simulink model "smo_pmsm"  (R2014a)
settings: Solver=ode45  StartTime=0.0  StopTime=0.5  RelTol=1e-3
InitFcn:
  | parameter
undefined symbols (not defined in the file): DiscIntNeverNeededParam, fc1, K, ki_i, ki_pll, ki_v, kp_i, kp_pll, kp_v, L, powergui, R, sigbuilder_block, Threshold, TS, Vdc, wc
libraries: powerlib x3, simulink x2, AC6DriveInternalModels x1
Description:
  | parameter.m;
settings Model: Creator=jzj  LastModifiedBy=jzj
settings ModelReferenceCC: ModelDependencies=parameter.m;

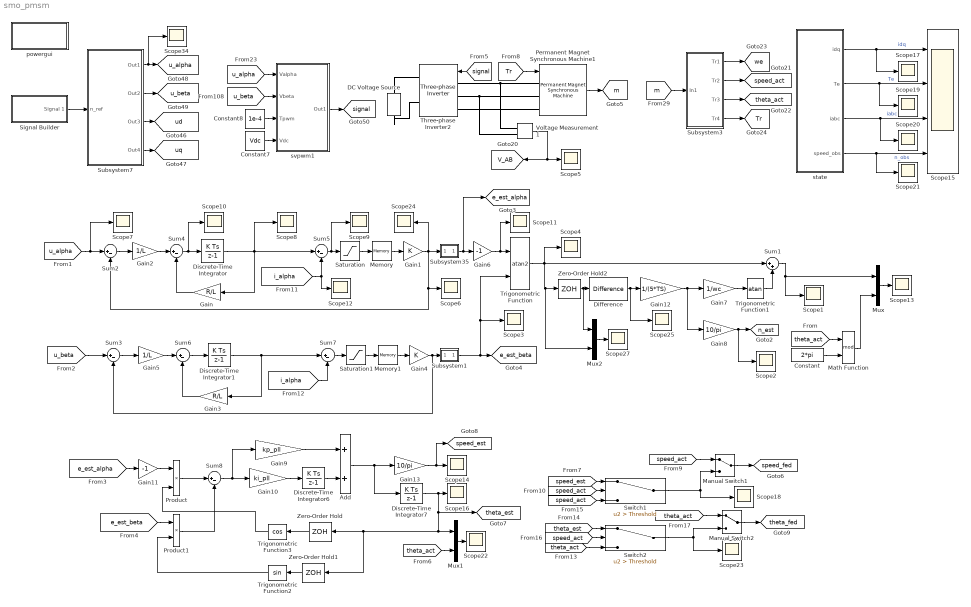
== system smo_pmsm ==
  Add : Sum
  Constant : Constant  Value=2*pi
  Constant7 : Constant  Value=Vdc
  Constant8 : Constant  Value=1e-4
  DC Voltage Source : powerlib/Electrical Sources/DC Voltage Source  Amplitude=Vdc  Measurements=Voltage
  Difference : simulink/Discrete/Difference  ICPrevInput=0.0  InputProcessing=Inherited  OutMin=[]  OutMax=[]  OutDataType=fixdt(1, 16)  OutScaling=2^-10  DoSatur=off
  Discrete-Time Integrator{,1,6..7} (4 alike) : DiscreteIntegrator  SampleTime=-1  ICPrevOutput=DiscIntNeverNeededParam  ICPrevScaledInput=DiscIntNeverNeededParam
  Gain : Gain  Gain=R/L
  Gain1 : Gain  Gain=K
  Gain10 : Gain  Gain=ki_pll
  Gain11 : Gain  Gain=-1
  Gain12 : Gain  Gain=1/(5*TS)
  Gain13 : Gain  Gain=10/pi
  Gain2 : Gain  Gain=1/L
  Gain3 : Gain  Gain=R/L
  Gain4 : Gain  Gain=K
  Gain5 : Gain  Gain=1/L
  Gain6 : Gain  Gain=-1
  Gain7 : Gain  Gain=1/wc
  Gain8 : Gain  Gain=10/pi
  Gain9 : Gain  Gain=kp_pll
  Manual Switch1 : ManualSwitch
  Manual Switch2 : ManualSwitch
  Math Function : Math  Operator=mod  SaturateOnIntegerOverflow=on
  Memory : Memory  InheritSampleTime=on
  Memory1 : Memory  InheritSampleTime=on
  Mux : Mux  Inputs=2
  Mux1 : Mux  Inputs=2
  Mux2 : Mux  Inputs=2
  Permanent Magnet Synchronous Machine1 : powerlib/Machines/Permanent Magnet Synchronous Machine  NbPhases=3  FluxDistribution=Sinusoidal  RotorType=Round  MechanicalLoad=Torque Tm  PresetModel=No  ShowDetailedParameters=on  MeasurementBus=off  Resistance=0.8  Inductance=0  dqInductances=[0.01,0.02]  La=0.0012  MachineConstant=Voltage Constant (V_peak L-L / krpm)  Flux=0.003308  VoltageCst=2.4  TorqueCst=0.019848  Flat=0  Mechanical=[0.0001,0,4]  PolePairs=3  InitialConditions=[0,0, 0,0]  InitialConditions5ph=[0 0 0 0 0 0]  TsPowergui=0  TsBlock=-1  RefAngle=Aligned with phase A axis (original Park)
      link override From: GotoTag=tp24d3e2ed_e96a_4fb0_a076_5c3b1daf5e05
      settings: AttributesFormatString=\n
  Product : Product
  Product1 : Product
  Saturation : Saturate  UpperLimit=5  LowerLimit=-5
  Saturation1 : Saturate  UpperLimit=5  LowerLimit=-5
  Scope{1..14,16..25,27,34} (26 alike) : Scope
      Scope1 settings: YMin=-700  YMax=700  SaveName=ScopeData7
      Scope10 settings: YMin=-700  YMax=700  SaveName=ScopeData24
      Scope11 settings: YMin=-700  YMax=700  SaveName=ScopeData25
      Scope12 settings: YMin=-700  YMax=700  SaveName=ScopeData31
      Scope13 settings: YMin=-700  YMax=700  SaveName=ScopeData32
      Scope14 settings: YMin=-700  YMax=700  SaveName=ScopeData33
      Scope16 settings: YMin=-700  YMax=700  SaveName=ScopeData34
      Scope17 settings: YMin=-700  YMax=700  SaveName=ScopeData18
      Scope18 settings: YMin=-700  YMax=700  SaveName=ScopeData35
      Scope19 settings: YMin=-700  YMax=700  SaveName=ScopeData19
      Scope2 settings: YMin=-700  YMax=700  SaveName=ScopeData10
      Scope20 settings: YMin=-700  YMax=700
      Scope21 settings: TimeRange=3  YMin=4200  YMax=5500  SaveName=ScopeData4
      Scope22 settings: YMin=-700  YMax=700  SaveName=ScopeData36
      Scope23 settings: YMin=-700  YMax=700  SaveName=ScopeData39
      Scope24 settings: YMin=-700  YMax=700  SaveName=ScopeData40
      Scope25 settings: YMin=-700  YMax=700  SaveName=ScopeData41
      Scope27 settings: YMin=-700  YMax=700  SaveName=ScopeData43
      Scope3 settings: YMin=-700  YMax=700  SaveName=ScopeData11
      Scope34 settings: YMin=-700  YMax=700  SaveName=ScopeData38
      Scope4 settings: YMin=-700  YMax=700  SaveName=ScopeData13
      Scope5 settings: YMin=-700  YMax=700  SaveName=ScopeData78
      Scope6 settings: YMin=-700  YMax=700  SaveName=ScopeData14
      Scope7 settings: YMin=-700  YMax=700  SaveName=ScopeData15
      Scope8 settings: YMin=-700  YMax=700  SaveName=ScopeData16
      Scope9 settings: YMin=-700  YMax=700  SaveName=ScopeData17
  Scope15 : Scope  NumInputPorts=4
      settings: TimeRange=1.5  YMin=-17.5~-5~-80~-400  YMax=15~35~60~900  SaveName=ScopeData20
  Signal Builder : Subsystem  Tag=STV Subsys  LoadFcn=sigbuilder_block('load');  StartFcn=sigbuilder_block('start');  StopFcn=sigbuilder_block('stop');  ClipboardFcn=sigbuilder_block('clipboard');  mask(Sigbuilder block){}
      mask help: Simulink:masks:SigbuilderBlock_MD
      mask init:
      | if ~strcmp(get_param(bdroot(gcbh),'SimulationStatus'),'stopped') tuvar = sigbuilder_block('maskInit'); end
      settings: CopyFcn=sigbuilder_block('copy');  DeleteFcn=sigbuilder_block('delete');  ModelCloseFcn=sigbuilder_block('modelClose');  PreSaveFcn=sigbuilder_block('preSave');  PauseFcn=sigbuilder_block('pause');  ContinueFcn=sigbuilder_block('continue');  NameChangeFcn=sigbuilder_block('namechange');  OpenFcn=sigbuilder_block('open',[497.25 145.5 550.5 399.75 ]);  CloseFcn=sigbuilder_block('close');
      mask Display: plot(0, 0, 100, 100,[2, 2, 32, 32, 2], [68, 8, 8, 68, 68],[32, 2], [38, 38], [32, 19, 2],[53, 60, 44], [32, 17, 17, 2],[16, 16, 31, 31]);txt = getActiveGroup(gcbh);text(2, 100, txt,'verticalAlignment', 'top');
  Subsystem1 : Subsystem
  Subsystem3 : Subsystem
  Subsystem35 : Subsystem
  Subsystem7 : Subsystem
  Sum1 : Sum  Inputs=|++
  Sum{2..8} (7 alike) : Sum  Inputs=|+-
  Switch1 : Switch  Criteria=u2 > Threshold  Threshold=Threshold
  Switch2 : Switch  Criteria=u2 > Threshold  Threshold=Threshold
  Three-phase Inverter2 : AC6DriveInternalModels/Three-phase Inverter  Arms=3  SnubberResistance=5000  SnubberCapacitance=inf  Device=IGBT / Diodes  Ron=1e-3  Lon=0  ForwardVoltages=[0.8,0.8]  ForwardVoltage=0  GTOparameters=[0,0]  IGBTParameters=[1e-6,2e-6]  Measurements=All voltages and currents  converterType=Inverter  SourceFrequency=60  dqInductances=[8.5e-3,8.5e-3]  Flux=0.175  Resistance=0.2  p=4
  Trigonometric Function : Trigonometry  Operator=atan2
  Trigonometric Function1 : Trigonometry  Operator=atan
  Trigonometric Function2 : Trigonometry
  Trigonometric Function3 : Trigonometry  Operator=cos
  Voltage Measurement1 : powerlib/Measurements/Voltage Measurement  PhasorSimulation=off  OutputType=Complex  PSBequivalent=0
  Zero-Order Hold : ZeroOrderHold  SampleTime=TS
  Zero-Order Hold1 : ZeroOrderHold  SampleTime=TS
  Zero-Order Hold2 : ZeroOrderHold  SampleTime=5*TS
  powergui : Subsystem  Priority=1  AncestorBlock=powerlib/powergui  InitFcn=powergui( 'InitFcn_Callback' , gcb , 0 , [ ] );  StopFcn=powergui( 'StopFcn_Callback' , gcb , 0 , [ ] );  mask(PSB option menu block){SimulationMode=Discrete, SolverType=Tustin, SampleTime=1e-6, frequency=60, SPID=off, DisableSnubberDevices=off, DisableRonSwitches=off, DisableVfSwitches=off, SwTol=0, Interpol=off, DisplayEquations=off, Ts=100, methode=off, frequencyindice=0, Pbase=100e6, ErrMax=1e-4, Iterations=50, UnitsV=kV, UnitsW=MW, FunctionMessages=off, echomessages=off, HookPort=off, EnableUseOfTLC=off, x0status=blocks, RestoreLinks=warning, ResistiveCurrentMeasurement=off, Frange=[0:2:500], Ylog=off, Xlog=on, ShowGrid=off, save=off, variable=ZData, structure=iabc1, ZoomFFT=off, StartTime=2.2, cycles=50, DisplayStyle=1, fundamental=200, FreqAxis=on, MaxFrequency=500, frequencyindicesteady=1, RmsSteady=1, display=off}
      mask prompts: SimulationMode "Simulation type:"; SolverType "Solver type:"; SampleTime "Sample time (s):"; frequency "Phasor frequency (Hz):"; SPID "Enable use of ideal switching devices"; DisableSnubberDevices "Disable snubbers in switching devices"; DisableRonSwitches "Disable On resistance in switching devices (Ron=0)"; DisableVfSwitches "Disable Forward voltage in switching devices (Vf=0)"; SwTol "Switch tolerance"; Interpol "Interpolate"; DisplayEquations "Display circuit differential equations"; Ts "Old Ts setting (OBSOLETE)"; methode "Phasor simulation (OBSOLETE)"; frequencyindice "Load flow frequency (Hz):"; Pbase "Base power Pbase (VA):"; ErrMax "PQ tolerance (pu):"; Iterations "Max iterations:"; UnitsV "Voltage units"; UnitsW "Power units"; FunctionMessages "Disable SimPowerSystems warnings"; echomessages "Display SimPowerSystems compilation messages"; HookPort "Add a hook port to the powergui block"; EnableUseOfTLC "Use TLC file when in Accelerator Simulation Mode and for code generation"; x0status "Start simulation with initial electrical states from:"; RestoreLinks "Restore disabled links of SimPowerSystems blocks:"; ResistiveCurrentMeasurement "Use non ideal current measurement blocks (1e-4Ohm internal resistance)"; Frange "Frequency Range"; Ylog "Log impedance"; Xlog "log Frequency"; ShowGrid "grid"; save "Save Data To Workspace"; variable "Variable Name"; structure "Structure Name (PSBFFTSCOPE)"; ZoomFFT "ZoomFFT (PSBFFTSCOPE)"; StartTime "Start Time (PSBFFTSCOPE)"; cycles "Cycles (PSBFFTSCOPE)"; DisplayStyle "Display style (PSBFFTSCOPE)"; fundamental "Fundamental (PSBFFTSCOPE)"; FreqAxis "Frequency Axis (PSBFFTSCOPE)"; MaxFrequency "Max Frequency (PSBFFTSCOPE)"; frequencyindicesteady "Frequency indice (STEADYSTATE)"; RmsSteady "RMS display (STEADYSTATE)"; display "Display Results"
      mask help: Set simulation type, simulation parameters, and preferences
      mask init:
      | message = powergui('MaskInitialization',gcb,SimulationMode,SampleTime);
      settings: CopyFcn=powergui( 'Copy_Callback' , gcb , 0 , [ ] );  ModelCloseFcn=powergui( 'CloseButton_Callback' , gcb , [ ] , [ ] );  NameChangeFcn=powergui( 'NameChangeFcn_Callback' , gcb , 0 , [ ] );  OpenFcn=powergui(gcb,'Open')
      settings: DeleteFcn=|
      | % see geck 675031 powergui( 'Copy_Callback' , gcb , 1 , [ ] );
      | 
      | powergui( 'CloseButton_Callback' , gcb , [ ] , [ ] );
      settings: PreSaveFcn=|
      | powergui( 'PreSaveFcn_Callback' , gcb , [ ] , [ ] );
      | powergui( 'CloseButton_Callback' , gcb , [ ] , [ ] );
      mask Help: helpview(psbhelp)
      mask TypeOptions SimulationMode: Continuous | Discrete | Phasor
      mask Callback SimulationMode: powergui('SimulationType',[],[],gcb);
      mask TypeOptions SolverType: Tustin | Backward Euler
      mask Callback SPID: powergui('SPID',[],[],gcb);
      mask TypeOptions UnitsV: V | kV
      mask TypeOptions UnitsW: W | kW | MW
      mask Callback HookPort: powergui('HookPort',[],[],gcb);
      mask TypeOptions x0status: blocks | steady | zero
      mask TypeOptions RestoreLinks: yes | warning | no
      mask Display: color('blue'),disp(message)
  state : Subsystem
  svpwm1 : Subsystem
  tag scope: Tr=global, V_AB=global, e_est_alpha=global, e_est_beta=global, m=global, n_est=global, signal=global, speed_act=global, speed_est=global, speed_fed=global, theta_act=global, theta_est=global, theta_fed=global, u_alpha=global, u_beta=global, ud=global, uq=global, we=global
  wires:
  Subsystem7/1(Out1) -> [u_alpha], Scope34/1
  Subsystem7/2(Out2) -> [u_beta]
  Subsystem7/3(Out3) -> [ud]
  Subsystem7/4(Out4) -> [uq]
  Constant8/1 -> svpwm1/3(Tpwm)
  Constant7/1 -> svpwm1/4(Vdc)
  svpwm1/1(Out1) -> [signal]
  [u_alpha] -> svpwm1/1(Valpha)
  [u_beta] -> svpwm1/2(Vbeta)
  [signal] -> Three-phase Inverter2/1
  [Tr] -> Permanent Magnet Synchronous Machine1/1
  Permanent Magnet Synchronous Machine1/1 -> [m]
  Voltage Measurement1/1 -> [V_AB], Scope5/1
  [m] -> Subsystem3/1(In1)
  Subsystem3/1(Tr1) -> [we]
  Subsystem3/2(Tr2) -> [speed_act]
  Subsystem3/3(Tr3) -> [theta_act]
  Subsystem3/4(Tr4) -> [Tr]
  state/1(idq) -> Scope15/1, Scope17/1  "idq"
  state/2(Te) -> Scope15/2, Scope19/1  "Te"
  state/3(iabc) -> Scope15/3, Scope20/1  "iabc"
  state/4(speed_obs) -> Scope15/4, Scope21/1  "n_obs"
  Signal Builder/1(Signal 1) -> Subsystem7/1(n_ref)
  [u_beta] -> Sum3/1
  [u_alpha] -> Scope7/1, Sum2/1
  Sum2/1 -> Gain2/1
  Sum4/1 -> Scope10/1, Discrete-Time Integrator/1
  Gain/1 -> Sum4/2
  Discrete-Time Integrator/1 -> Scope8/1, Sum5/1, Gain/1
  [i_alpha] -> Scope12/1, Sum5/2
  Sum5/1 -> Scope9/1, Saturation/1
  Saturation/1 -> Memory/1
  Memory/1 -> Gain1/1
  Gain2/1 -> Sum4/1
  Sum6/1 -> Discrete-Time Integrator1/1
  Gain3/1 -> Sum6/2
  Discrete-Time Integrator1/1 -> Gain3/1, Sum7/1
  [i_alpha] -> Sum7/2
  Sum7/1 -> Saturation1/1
  Saturation1/1 -> Memory1/1
  Memory1/1 -> Gain4/1
  Gain5/1 -> Sum6/1
  Sum3/1 -> Gain5/1
  Gain1/1 -> Subsystem35/1(fil), Scope24/1, Scope6/1, Sum2/2
  Gain4/1 -> Subsystem1/1(fil), Sum3/2
  Subsystem35/1(ter) -> [e_est_alpha], Gain6/1
  Gain6/1 -> Scope11/1, Trigonometric Function/1
  Subsystem1/1(ter) -> [e_est_beta], Scope3/1, Trigonometric Function/2
  Trigonometric Function/1 -> Mux2/2, Zero-Order Hold2/1, Sum1/1, Scope4/1
  Gain7/1 -> Trigonometric Function1/1
  Trigonometric Function1/1 -> Sum1/2
  Sum1/1 -> Scope1/1, Mux/1
  Gain8/1 -> Scope2/1, [n_est]
  [theta_act] -> Math Function/1
  Constant/1 -> Math Function/2
  Math Function/1 -> Mux/2
  Mux/1 -> Scope13/1
  Discrete-Time Integrator6/1 -> Add/2
  Gain9/1 -> Add/1
  Gain10/1 -> Discrete-Time Integrator6/1
  [e_est_alpha] -> Gain11/1
  Gain11/1 -> Product/1
  [e_est_beta] -> Product1/1
  Product/1 -> Sum8/1
  Product1/1 -> Sum8/2
  Sum8/1 -> Gain9/1, Gain10/1
  Trigonometric Function3/1 -> Product/2
  Trigonometric Function2/1 -> Product1/2
  Discrete-Time Integrator7/1 -> [theta_est], Mux1/1, Zero-Order Hold1/1, Zero-Order Hold/1, Scope16/1
  Zero-Order Hold/1 -> Trigonometric Function3/1
  Zero-Order Hold1/1 -> Trigonometric Function2/1
  [theta_act] -> Mux1/2
  Mux1/1 -> Scope22/1
  Add/1 -> Discrete-Time Integrator7/1, Gain13/1
  Gain13/1 -> [speed_est], Scope14/1
  Manual Switch1/1 -> [speed_fed]
  [speed_act] -> Manual Switch1/1
  Switch1/1 -> Scope18/1, Manual Switch1/2
  [speed_act] -> Switch1/2
  [speed_act] -> Switch1/3
  [speed_est] -> Switch1/1
  [theta_est] -> Switch2/1
  [speed_act] -> Switch2/2
  [theta_act] -> Switch2/3
  Manual Switch2/1 -> [theta_fed]
  [theta_act] -> Manual Switch2/1
  Switch2/1 -> Manual Switch2/2, Scope23/1
  Zero-Order Hold2/1 -> Mux2/1, Difference/1
  Difference/1 -> Scope25/1, Gain12/1
  Gain12/1 -> Gain8/1, Gain7/1
  Mux2/1 -> Scope27/1
  connections:
  Three-phase Inverter2/LConn1 -- Permanent Magnet Synchronous Machine1/LConn1 -- Voltage Measurement1/LConn1
  Voltage Measurement1/LConn2 -- Permanent Magnet Synchronous Machine1/LConn2 -- Three-phase Inverter2/LConn2
  Permanent Magnet Synchronous Machine1/LConn3 -- Three-phase Inverter2/LConn3
  DC Voltage Source/RConn1 -- Three-phase Inverter2/RConn1
  DC Voltage Source/LConn1 -- Three-phase Inverter2/RConn2

== system smo_pmsm/Signal Builder ==
  Demux : Demux  Tag=STV Demux  Outputs=1
  FromWs : FromWorkspace  Tag=STV FromWs  VariableName=tuvar  SampleTime=0
      SigBuilderData=|
      | common.afterFinalStr = 'Extrapolate'
      | common.sampleTime = 0
      | dataSet.timeRange = [0 10]
      | dataSet.name = 'Group 1'
      | sbobj.Groups.Name = 'Group 1'
      | sbobj.Groups.Signals.Name = 'Signal 1'
      | sbobj.Groups.Signals.XData = [0 0.2 4 6 10]
      | sbobj.Groups.Signals.YData = [0 2000 2000 2000 2000]
  Signal 1 : Outport  Tag=STV Outport
  wires:
  Demux/1 -> Signal 1/1
  FromWs/1 -> Demux/1

== system smo_pmsm/Subsystem1 ==
  fil : Inport
  Low pass filter : DiscreteTransferFcn  Numerator=[1-exp(-2*pi*fc1*TS)]  Denominator=[1 -exp(-2*pi*fc1*TS)]  SampleTime=TS
  ter : Outport
  wires:
  Low pass filter/1 -> ter/1
  fil/1 -> Low pass filter/1

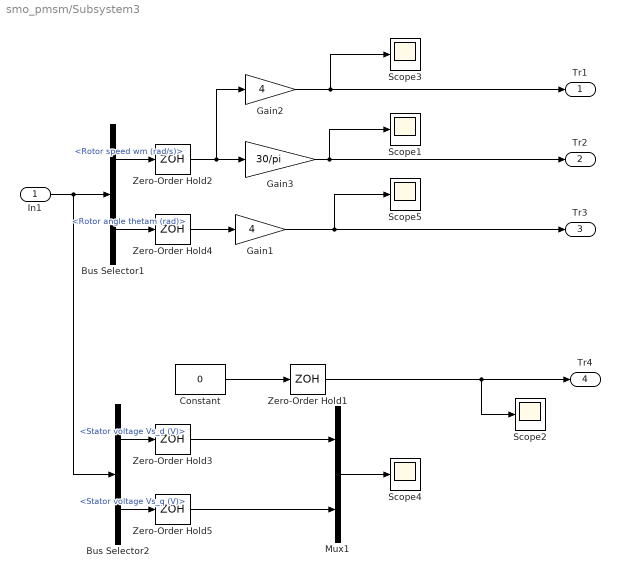
== system smo_pmsm/Subsystem3 ==
  In1 : Inport
  Bus Selector1 : BusSelector  OutputSignals=Rotor speed wm (rad/s),Rotor angle thetam (rad)
  Bus Selector2 : BusSelector  OutputSignals=Stator voltage Vs_d (V),Stator voltage Vs_q (V)
  Constant : Constant  Value=0
  Gain1 : Gain  Gain=4
  Gain2 : Gain  Gain=4
  Gain3 : Gain  Gain=30/pi
  Mux1 : Mux  Inputs=2
  Scope{1..5} (5 alike) : Scope
      Scope1 settings: YMin=-500  YMax=700  SaveName=ScopeData9
      Scope2 settings: YMin=-25  YMax=400  SaveName=ScopeData149
      Scope3 settings: YMin=185.5  YMax=191.5  SaveName=ScopeData79
      Scope4 settings: YMin=-25  YMax=400  SaveName=ScopeData88
      Scope5 settings: YMin=195  YMax=202.5  SaveName=ScopeData90
  Zero-Order Hold{1..5} (5 alike) : ZeroOrderHold  SampleTime=TS
  Tr1 : Outport
  Tr2 : Outport  Port=2
  Tr3 : Outport  Port=3
  Tr4 : Outport  Port=4
  wires:
  Zero-Order Hold5/1 -> Mux1/2
  Zero-Order Hold3/1 -> Mux1/1
  Constant/1 -> Zero-Order Hold1/1
  In1/1 -> Bus Selector1/1, Bus Selector2/1
  Bus Selector1/1 -> Zero-Order Hold2/1  "<Rotor speed wm (rad/s)>"
  Bus Selector1/2 -> Zero-Order Hold4/1  "<Rotor angle thetam (rad)>"
  Zero-Order Hold2/1 -> Gain2/1, Gain3/1
  Zero-Order Hold4/1 -> Gain1/1
  Gain2/1 -> Tr1/1, Scope3/1
  Gain3/1 -> Scope1/1, Tr2/1
  Zero-Order Hold1/1 -> Scope2/1, Tr4/1
  Bus Selector2/1 -> Zero-Order Hold3/1  "<Stator voltage Vs_d (V)>"
  Bus Selector2/2 -> Zero-Order Hold5/1  "<Stator voltage Vs_q (V)>"
  Gain1/1 -> Tr3/1, Scope5/1
  Mux1/1 -> Scope4/1

== system smo_pmsm/Subsystem35 ==
  fil : Inport
  Low pass filter : DiscreteTransferFcn  Numerator=[1-exp(-2*pi*fc1*TS)]  Denominator=[1 -exp(-2*pi*fc1*TS)]  SampleTime=TS
  ter : Outport
  wires:
  fil/1 -> Low pass filter/1
  Low pass filter/1 -> ter/1

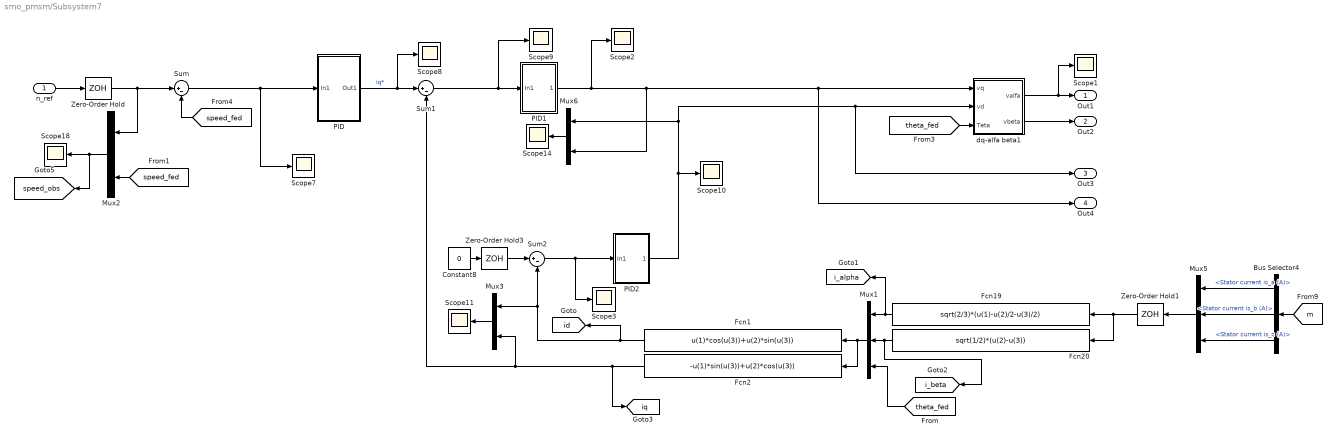
== system smo_pmsm/Subsystem7 ==
  n_ref : Inport
  Bus Selector4 : BusSelector  OutputSignals=Stator current is_a (A),Stator current is_b (A),Stator current is_c (A)
  Constant8 : Constant  Value=0
  Fcn1 : Fcn  Expr=u(1)*cos(u(3))+u(2)*sin(u(3))
  Fcn19 : Fcn  Expr=sqrt(2/3)*(u(1)-u(2)/2-u(3)/2)
  Fcn2 : Fcn  Expr=-u(1)*sin(u(3))+u(2)*cos(u(3))
  Fcn20 : Fcn  Expr=sqrt(1/2)*(u(2)-u(3))
  Mux1 : Mux  Inputs=3
  Mux2 : Mux  Inputs=2
  Mux3 : Mux  Inputs=2
  Mux5 : Mux  Inputs=3
  Mux6 : Mux  Inputs=2
  PID : Subsystem
  PID1 : Subsystem
  PID2 : Subsystem
  Scope{1..3,7..11,14,18} (10 alike) : Scope
      Scope1 settings: SaveName=ScopeData37
      Scope10 settings: SaveName=ScopeData30
      Scope11 settings: TimeRange=1.7  YMin=-15  YMax=17.5  SaveName=ScopeData71
      Scope14 settings: TimeRange=1.7  YMin=-15  YMax=17.5  SaveName=ScopeData106
      Scope18 settings: TimeRange=0.01073731461302402  YMin=996.9949713569969  YMax=1006.526183941498  SaveName=ScopeData21
      Scope2 settings: SaveName=ScopeData22
      Scope3 settings: SaveName=ScopeData23
      Scope7 settings: SaveName=ScopeData26
      Scope8 settings: SaveName=ScopeData28
      Scope9 settings: SaveName=ScopeData29
  Sum : Sum  Inputs=|+-
  Sum1 : Sum  Inputs=|+-
  Sum2 : Sum  Inputs=|+-
  Zero-Order Hold : ZeroOrderHold  SampleTime=TS
  Zero-Order Hold1 : ZeroOrderHold  SampleTime=TS
  Zero-Order Hold3 : ZeroOrderHold  SampleTime=TS
  dq-alfa beta1 : Subsystem
  Out1 : Outport
  Out2 : Outport  Port=2
  Out3 : Outport  Port=3
  Out4 : Outport  Port=4
  tag scope: i_alpha=global, i_beta=global, id=global, iq=global, speed_obs=global
  wires:
  Sum1/1 -> PID1/1(In1), Scope9/1
  Sum2/1 -> Scope3/1, PID2/1(In1)
  Mux2/1 -> [speed_obs], Scope18/1
  Sum/1 -> PID/1(In1), Scope7/1
  Constant8/1 -> Zero-Order Hold3/1
  Zero-Order Hold3/1 -> Sum2/1
  [theta_fed] -> dq-alfa beta1/3(Teta)
  [speed_fed] -> Mux2/2
  Zero-Order Hold/1 -> Sum/1, Mux2/1
  n_ref/1 -> Zero-Order Hold/1
  Mux3/1 -> Scope11/1
  PID/1(Out1) -> Scope8/1, Sum1/1  "iq*"
  [speed_fed] -> Sum/2
  PID2/1(Out1) -> Scope10/1, Mux6/1, dq-alfa beta1/2(vd), Out3/1
  PID1/1(Out1) -> Mux6/2, dq-alfa beta1/1(vq), Out4/1, Scope2/1
  dq-alfa beta1/1(valfa) -> Out1/1, Scope1/1
  dq-alfa beta1/2(vbeta) -> Out2/1
  Fcn1/1 -> Mux3/1, Sum2/2, [id]
  Fcn2/1 -> [iq], Sum1/2, Mux3/2
  Mux6/1 -> Scope14/1
  [m] -> Bus Selector4/1
  Bus Selector4/2 -> Mux5/2  "<Stator current is_b (A)>"
  Bus Selector4/3 -> Mux5/3  "<Stator current is_c (A)>"
  Bus Selector4/1 -> Mux5/1  "<Stator current is_a (A)>"
  Mux5/1 -> Zero-Order Hold1/1
  Fcn19/1 -> [i_alpha], Mux1/1
  Fcn20/1 -> [i_beta], Mux1/2
  [theta_fed] -> Mux1/3
  Mux1/1 -> Fcn2/1, Fcn1/1
  Zero-Order Hold1/1 -> Fcn20/1, Fcn19/1

== system smo_pmsm/powergui ==
  note: Graphical user interface for the analysis of  SimPowerSystems circuits.
      | Place the Powergui block in the top-level of your model and double-click
      | on it to open the GUI.
  EquivalentModel1 : Subsystem
      mask init:
      | S  = GetDataForEquivalentModel('Discrete',gcbh);
      mask Display:
      | color('red')
      | disp('EQUIVALENT CIRCUIT\nDiscrete')
  Ground : Ground
  Terminator : Terminator
  wires:
  Ground/1 -> Terminator/1

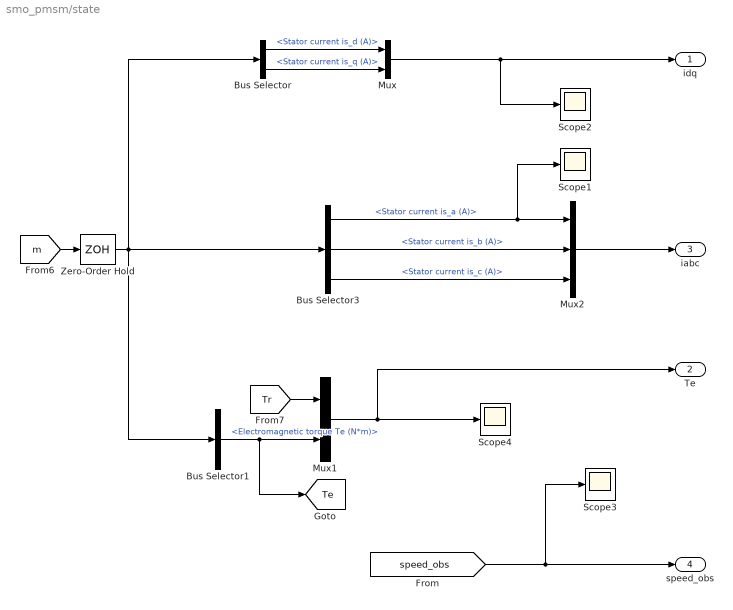
== system smo_pmsm/state ==
  Bus Selector : BusSelector  OutputSignals=Stator current is_d (A),Stator current is_q (A)
  Bus Selector1 : BusSelector  OutputSignals=Electromagnetic torque Te (N*m)
  Bus Selector3 : BusSelector  OutputSignals=Stator current is_a (A),Stator current is_b (A),Stator current is_c (A)
  Mux : Mux  Inputs=2
  Mux1 : Mux  Inputs=2
  Mux2 : Mux  Inputs=3
  Scope{1..4} (4 alike) : Scope
      Scope1 settings: TimeRange=0.7000000000000001  YMin=-4  YMax=8  SaveName=iabc
      Scope2 settings: TimeRange=0.7000000000000001  YMin=-2  YMax=18  SaveName=iabc1
      Scope3 settings: TimeRange=0.7000000000000001  YMin=1700  YMax=1712  SaveName=iabc2
      Scope4 settings: TimeRange=0.7000000000000001  YMin=-4  YMax=8  SaveName=iabc3
  Zero-Order Hold : ZeroOrderHold  SampleTime=TS
  idq : Outport
  Te : Outport  Port=2
  iabc : Outport  Port=3
  speed_obs : Outport  Port=4
  tag scope: Te=global
  wires:
  Bus Selector/1 -> Mux/1  "<Stator current is_d (A)>"
  Bus Selector/2 -> Mux/2  "<Stator current is_q (A)>"
  Bus Selector3/1 -> Mux2/1, Scope1/1  "<Stator current is_a (A)>"
  Bus Selector3/3 -> Mux2/3  "<Stator current is_c (A)>"
  Bus Selector3/2 -> Mux2/2  "<Stator current is_b (A)>"
  Bus Selector1/1 -> [Te], Mux1/2  "<Electromagnetic torque Te (N*m)>"
  [m] -> Zero-Order Hold/1
  [Tr] -> Mux1/1
  Mux/1 -> Scope2/1, idq/1
  Zero-Order Hold/1 -> Bus Selector/1, Bus Selector1/1, Bus Selector3/1
  Mux2/1 -> iabc/1
  [speed_obs] -> Scope3/1, speed_obs/1
  Mux1/1 -> Scope4/1, Te/1

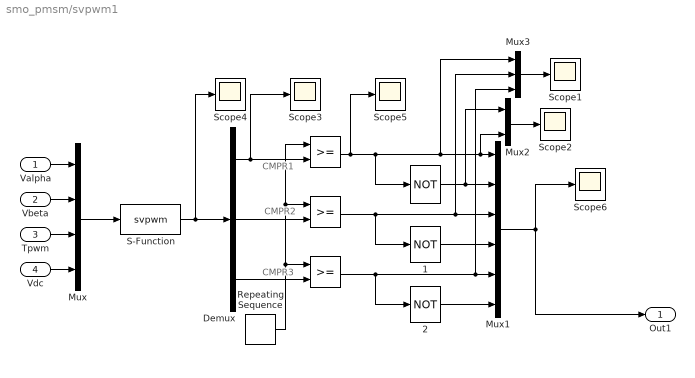
== system smo_pmsm/svpwm1 ==
  note: CMPR1
  note: CMPR2
  note: CMPR3
  Valpha : Inport
  Vbeta : Inport  Port=2
  Tpwm : Inport  Port=3
  Vdc : Inport  Port=4
  " " : RelationalOperator  ZeroCross=off
  "  " : RelationalOperator  OutDataTypeStr=boolean
  "   " : RelationalOperator  OutDataTypeStr=boolean
  "    " : Logic  Operator=NOT  Inputs=1  AllPortsSameDT=off  OutDataTypeStr=boolean
  "    1" : Logic  Operator=NOT  Inputs=1  AllPortsSameDT=off  OutDataTypeStr=boolean
  "    2" : Logic  Operator=NOT  Inputs=1  AllPortsSameDT=off  OutDataTypeStr=boolean
  Demux : Demux  Outputs=3
  Mux : Mux
  Mux1 : Mux  Inputs=6
  Mux2 : Mux  Inputs=2
  Mux3 : Mux  Inputs=3
  Repeating Sequence : simulink/Sources/Repeating Sequence  rep_seq_t=[0 0.00005 0.0001]  rep_seq_y=[0 0.00005 0]
  S-Function : S-Function  FunctionName=svpwm  EnableBusSupport=off
  Scope{1..6} (6 alike) : Scope
      Scope1 settings: TimeRange=1  YMin=-1  YMax=2  SaveName=ScopeData3
      Scope2 settings: TimeRange=0.2  YMin=-2.5e-006  YMax=5.25e-005  SaveName=ScopeData5
      Scope3 settings: TimeRange=0.2  YMin=-2.5e-006  YMax=5.25e-005
      Scope4 settings: TimeRange=0.2  YMin=-2.5e-006  YMax=5.25e-005  SaveName=ScopeData6
      Scope5 settings: TimeRange=0.2  YMin=-2.5e-006  YMax=5.25e-005  SaveName=ScopeData2
      Scope6 settings: TimeRange=0.2  YMin=-2.5e-006  YMax=5.25e-005  SaveName=ScopeData8
  Out1 : Outport
  wires:
  Demux/1 -> " "/2, Scope3/1
  Demux/2 -> "  "/2
  Demux/3 -> "   "/2
  "   "/1 -> "    2"/1, Mux1/5, Mux3/3
  "    "/1 -> Mux1/2, Mux2/1
  " "/1 -> Mux1/1, Mux2/2, Mux3/1, "    "/1, Scope5/1
  "  "/1 -> "    1"/1, Mux1/3, Mux3/2
  "    1"/1 -> Mux1/4
  "    2"/1 -> Mux1/6
  Repeating Sequence/1 -> "  "/1, " "/1, "   "/1
  S-Function/1 -> Demux/1, Scope4/1
  Valpha/1 -> Mux/1
  Vbeta/1 -> Mux/2
  Tpwm/1 -> Mux/3
  Vdc/1 -> Mux/4
  Mux3/1 -> Scope1/1
  Mux/1 -> S-Function/1
  Mux1/1 -> Out1/1, Scope6/1
  Mux2/1 -> Scope2/1

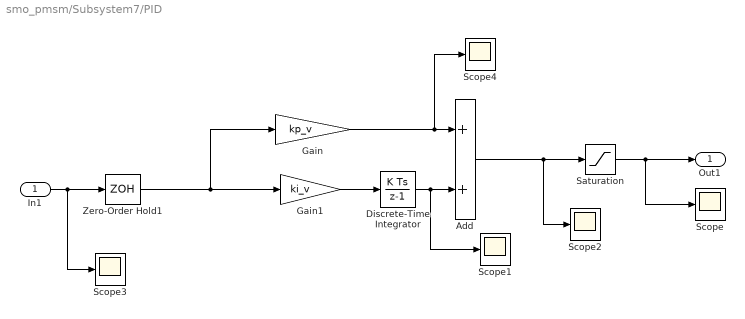
== system smo_pmsm/Subsystem7/PID ==
  In1 : Inport
  Add : Sum
  Discrete-Time Integrator : DiscreteIntegrator  InitialConditionSetting=State (most efficient)  SampleTime=-1  ICPrevOutput=DiscIntNeverNeededParam  ICPrevScaledInput=DiscIntNeverNeededParam
  Gain : Gain  Gain=kp_v
  Gain1 : Gain  Gain=ki_v
  Saturation : Saturate  UpperLimit=15  LowerLimit=-10
  Scope{,1..4} (5 alike) : Scope
      Scope settings: SaveName=ScopeData12
      Scope1 settings: SaveName=ScopeData27
      Scope2 settings: SaveName=ScopeData68
      Scope3 settings: SaveName=ScopeData69
      Scope4 settings: SaveName=ScopeData87
  Zero-Order Hold1 : ZeroOrderHold  SampleTime=TS
  Out1 : Outport
  wires:
  In1/1 -> Scope3/1, Zero-Order Hold1/1
  Gain/1 -> Scope4/1, Add/1
  Discrete-Time Integrator/1 -> Scope1/1, Add/2
  Add/1 -> Scope2/1, Saturation/1
  Saturation/1 -> Out1/1, Scope/1
  Gain1/1 -> Discrete-Time Integrator/1
  Zero-Order Hold1/1 -> Gain/1, Gain1/1

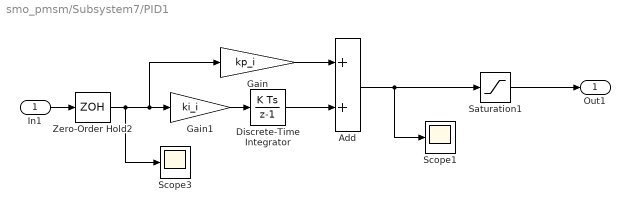
== system smo_pmsm/Subsystem7/PID1 ==
  In1 : Inport
  Add : Sum
  Discrete-Time Integrator : DiscreteIntegrator  InitialConditionSetting=State (most efficient)  SampleTime=-1  ICPrevOutput=DiscIntNeverNeededParam  ICPrevScaledInput=DiscIntNeverNeededParam
  Gain : Gain  Gain=kp_i
  Gain1 : Gain  Gain=ki_i
  Saturation1 : Saturate  UpperLimit=300  LowerLimit=-300
  Scope1 : Scope
      settings: SaveName=ScopeData64
  Scope3 : Scope
      settings: SaveName=ScopeData65
  Zero-Order Hold2 : ZeroOrderHold  SampleTime=TS
  Out1 : Outport
  wires:
  Saturation1/1 -> Out1/1
  Discrete-Time Integrator/1 -> Add/2
  Gain/1 -> Add/1
  Gain1/1 -> Discrete-Time Integrator/1
  In1/1 -> Zero-Order Hold2/1
  Add/1 -> Scope1/1, Saturation1/1
  Zero-Order Hold2/1 -> Scope3/1, Gain/1, Gain1/1

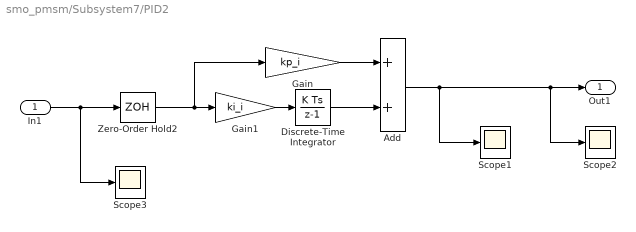
== system smo_pmsm/Subsystem7/PID2 ==
  In1 : Inport
  Add : Sum
  Discrete-Time Integrator : DiscreteIntegrator  InitialConditionSetting=State (most efficient)  SampleTime=-1  ICPrevOutput=DiscIntNeverNeededParam  ICPrevScaledInput=DiscIntNeverNeededParam
  Gain : Gain  Gain=kp_i
  Gain1 : Gain  Gain=ki_i
  Scope1 : Scope
      settings: YMin=-185  YMax=-115  SaveName=ScopeData67
  Scope2 : Scope
      settings: SaveName=ScopeData66
  Scope3 : Scope
      settings: SaveName=ScopeData70
  Zero-Order Hold2 : ZeroOrderHold  SampleTime=TS
  Out1 : Outport
  wires:
  Zero-Order Hold2/1 -> Gain1/1, Gain/1
  In1/1 -> Scope3/1, Zero-Order Hold2/1
  Gain1/1 -> Discrete-Time Integrator/1
  Gain/1 -> Add/1
  Discrete-Time Integrator/1 -> Add/2
  Add/1 -> Scope2/1, Out1/1, Scope1/1

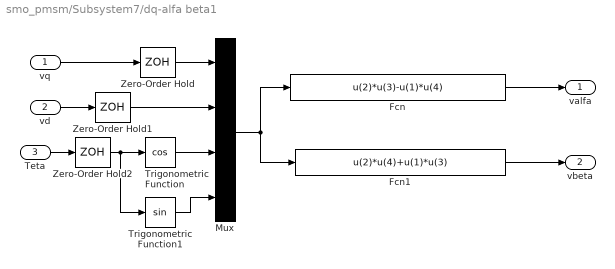
== system smo_pmsm/Subsystem7/dq-alfa beta1 ==
  vq : Inport
  vd : Inport  Port=2
  Teta : Inport  Port=3
  Fcn : Fcn  Expr=u(2)*u(3)-u(1)*u(4)
  Fcn1 : Fcn  Expr=u(2)*u(4)+u(1)*u(3)
  Mux : Mux
  Trigonometric Function : Trigonometry  Operator=cos
  Trigonometric Function1 : Trigonometry
  Zero-Order Hold : ZeroOrderHold  SampleTime=TS
  Zero-Order Hold1 : ZeroOrderHold  SampleTime=TS
  Zero-Order Hold2 : ZeroOrderHold  SampleTime=TS
  valfa : Outport
  vbeta : Outport  Port=2
  wires:
  Mux/1 -> Fcn/1, Fcn1/1
  Fcn/1 -> valfa/1
  Fcn1/1 -> vbeta/1
  Trigonometric Function/1 -> Mux/3
  Trigonometric Function1/1 -> Mux/4
  vq/1 -> Zero-Order Hold/1
  Zero-Order Hold/1 -> Mux/1
  vd/1 -> Zero-Order Hold1/1
  Zero-Order Hold1/1 -> Mux/2
  Teta/1 -> Zero-Order Hold2/1
  Zero-Order Hold2/1 -> Trigonometric Function/1, Trigonometric Function1/1

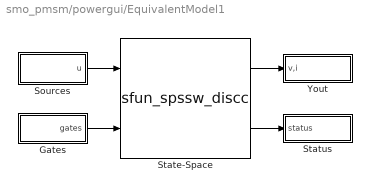
== system smo_pmsm/powergui/EquivalentModel1 ==
  Gates : Subsystem
  Sources : Subsystem
  State-Space : S-Function  FunctionName=sfun_spssw_discc  Parameters=S.Ts,S.A, S.B, S.C, S.D, S.x0, S.EnableUseOfTLC,S.SwitchResistance ,S.SwitchType, S.SwitchGateInitialValue, S.OutputsToResetToZero  EnableBusSupport=off
  Status : Subsystem
  Yout : Subsystem
  wires:
  Gates/1(gates) -> State-Space/2
  Sources/1(u) -> State-Space/1
  State-Space/2 -> Status/1(status)
  State-Space/1 -> Yout/1(v,i)

== system smo_pmsm/powergui/EquivalentModel1/Gates ==
  Mux : Mux  Inputs=1
  gates : Outport
  wires:
  Mux/1 -> gates/1
  [T52_5006_4458119330407] -> Mux/1

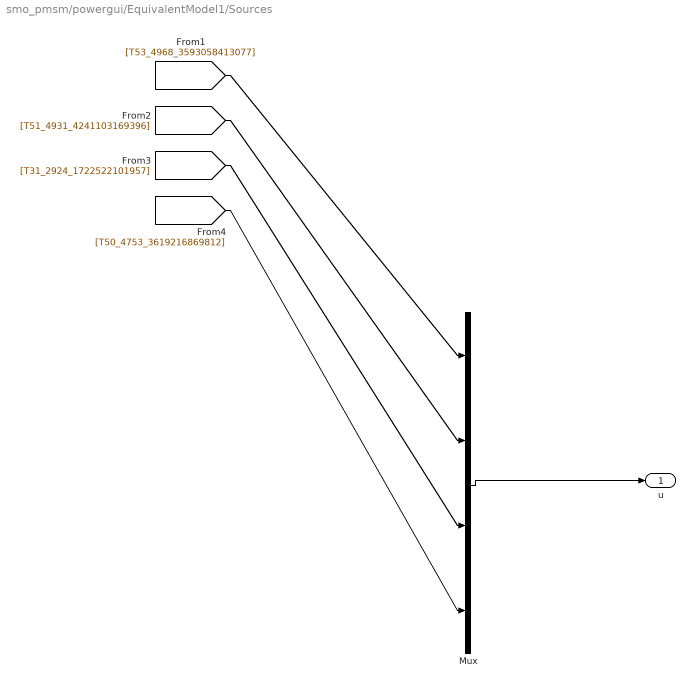
== system smo_pmsm/powergui/EquivalentModel1/Sources ==
  Mux : Mux  Inputs=[6 2 1 6]
  u : Outport
  wires:
  Mux/1 -> u/1
  [T53_4968_3593058413077] -> Mux/1
  [T51_4931_4241103169396] -> Mux/2
  [T31_2924_1722522101957] -> Mux/3
  [T50_4753_3619216869812] -> Mux/4

== system smo_pmsm/powergui/EquivalentModel1/Status ==
  status : Inport
  Demux : Demux  Outputs=1
  tag scope: T54_5241_5095670874902=global
  wires:
  status/1 -> Demux/1
  Demux/1 -> [T54_5241_5095670874902]

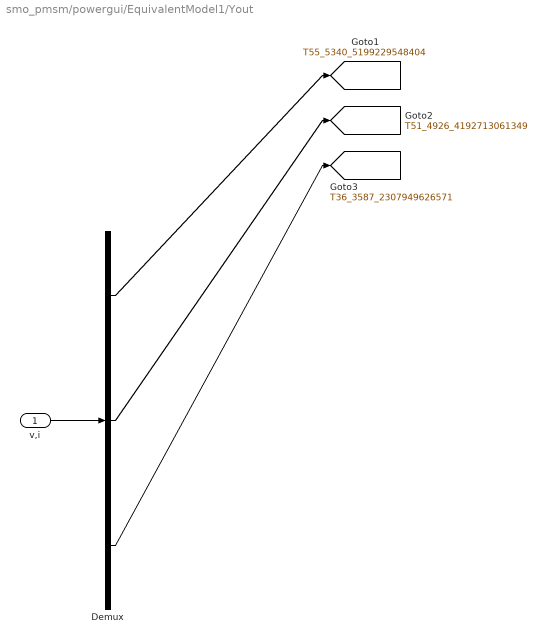
== system smo_pmsm/powergui/EquivalentModel1/Yout ==
  v,i : Inport
  Demux : Demux  Outputs=[6 2 1]
  tag scope: T36_3587_2307949626571=global, T51_4926_4192713061349=global, T55_5340_5199229548404=global
  wires:
  v,i/1 -> Demux/1
  Demux/1 -> [T55_5340_5199229548404]
  Demux/2 -> [T51_4926_4192713061349]
  Demux/3 -> [T36_3587_2307949626571]
